simulink model "star_measurement_model"  (R2025a)
settings: Solver=FixedStepAuto  StartTime=0.0  StopTime=5000  FixedStep=0.5  RelTol=1e-4
model mask{star=star}
model workspace (MAT data in the model file):
  star = 0
values from neighbouring files (symbols this model uses):
  m = size(A, 2)    [wheel_analysis.m]
  s = sign(h_bias)    [min_h.m]
  star_Ts = star.Ts    [orbit_params.m]
  Ts = 0.1    [orbit_params.m]    (also in untitled2.m = 0.005)
undefined symbols (not defined in the file or in its folder): earth, sigma_u, sigma_v
libraries: simulink x9, dspmathops x5, aerolibutil x4, utilities x2, simulink_extras x1
settings Model: ParameterArgumentNames=star  Creator=OlguPilav  LastModifiedBy=OlguPilav
settings DataIOCC: SaveOutput=off  SaveTime=off

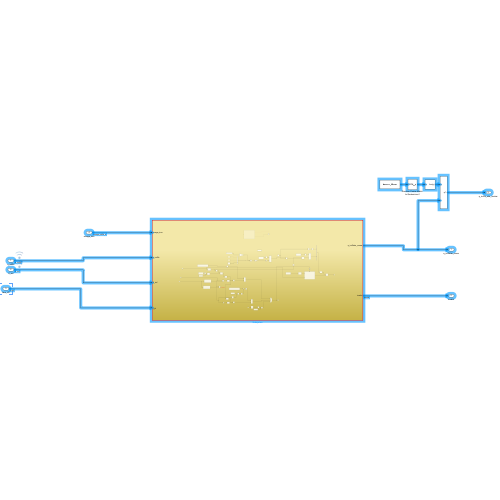
[thumbnail: Simulink's stored preview of the top-level diagram]
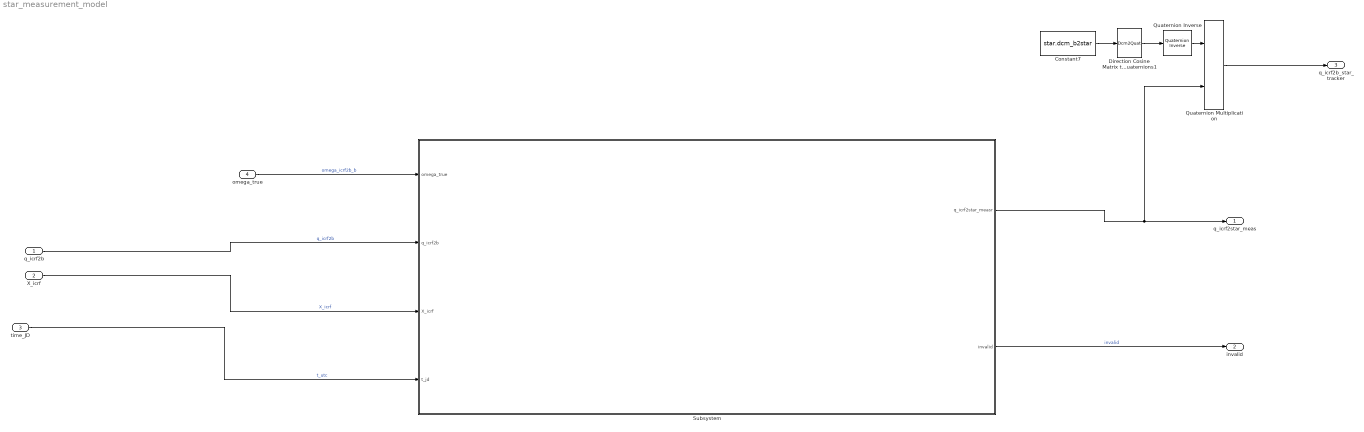
== system star_measurement_model ==
  q_icrf2b : Inport  OutDataTypeStr=double  PortDimensions=[4 1]  SampleTime=0
  X_icrf : Inport  Port=2  OutDataTypeStr=double  PortDimensions=3  SampleTime=0
  time_JD : Inport  Port=3  OutDataTypeStr=double  PortDimensions=1  SampleTime=0
  omega_true : Inport  Port=4  OutDataTypeStr=double  PortDimensions=3  SampleTime=0
  Constant7 : Constant  Value=star.dcm_b2star
  Direction Cosine Matrix to Quaternions1 : Dcm2Quat
  Quaternion Inverse : aerolibutil/Quaternion Inverse
  Quaternion Multiplication : aerolibutil/Quaternion Multiplication
  Subsystem : Subsystem  TreatAsAtomicUnit=on  SystemSampleTime=star_Ts
  q_icrf2star_meas : Outport  OutDataTypeStr=double  PortDimensions=4  SampleTime=[0.5,0]
  invalid : Outport  Port=2  OutDataTypeStr=boolean  PortDimensions=1  SampleTime=[0.5,0]
  q_icrf2b_star_tracker : Outport  Port=3  OutDataTypeStr=double  PortDimensions=4  SampleTime=[0.5,0]
  wires:
  q_icrf2b/1 -> Subsystem/2(q_icrf2b)  "q_icrf2b"
  X_icrf/1 -> Subsystem/3(X_icrf)  "X_icrf"
  time_JD/1 -> Subsystem/4(t_jd)  "t_utc"
  Subsystem/1(q_icrf2star_measr) -> q_icrf2star_meas/1, Quaternion Multiplication/2
  omega_true/1 -> Subsystem/1(omega_true)  "omega_icrf2b_b"
  Subsystem/2(invalid) -> invalid/1  "invalid"
  Quaternion Multiplication/1 -> q_icrf2b_star_tracker/1
  Constant7/1 -> Direction Cosine Matrix to Quaternions1/1
  Quaternion Inverse/1 -> Quaternion Multiplication/1
  Direction Cosine Matrix to Quaternions1/1 -> Quaternion Inverse/1

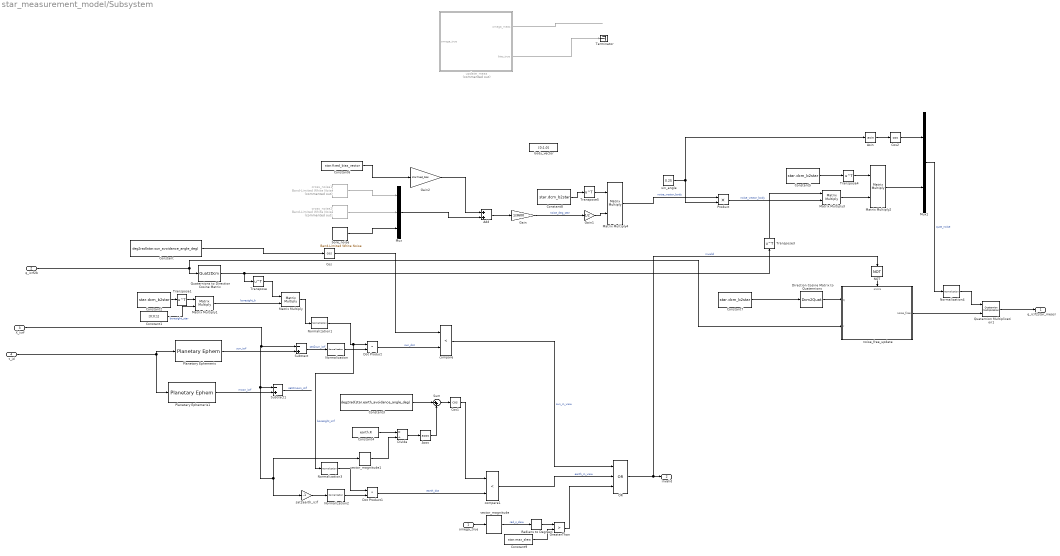
== system star_measurement_model/Subsystem ==
  omega_true : Inport
  q_icrf2b : Inport  Port=2
  X_icrf : Inport  Port=3
  t_jd : Inport  Port=4
  Acos : Trigonometry  Operator=acos
  Add : Sum
  Asin : Trigonometry  Operator=asin
  Constant : Constant  Value=deg2rad(star.sun_avoidance_angle_deg)
  Constant1 : Constant  Value=[0;0;1]
  Constant{2,5,7..8} (4 alike) : Constant  Value=star.dcm_b2star
  Constant3 : Constant  Value=deg2rad(star.earth_avoidance_angle_deg)
  Constant4 : Constant  Value=earth.R
  Constant6 : Constant  Value=star.fixed_bias_vector
  Constant9 : Constant  Value=star.max_slew
  Cos : Trigonometry  Operator=cos
  Cos1 : Trigonometry  Operator=cos
  Cos2 : Trigonometry  Operator=cos
  Direction Cosine Matrix to Quaternions : Dcm2Quat
  Divide : Product  Inputs=*/
  Dot Product : DotProduct  OutDataTypeStr=Inherit: Inherit via internal rule
  Dot Product1 : DotProduct  OutDataTypeStr=Inherit: Inherit via internal rule
  Gain : Gain  Gain=1/3600
  Gain1 : Gain  Gain=1/2
  Gain2 : Gain  Gain=star.fixed_bias
  GreaterThan : RelationalOperator  Operator=>  OutDataTypeStr=boolean  RndMeth=Simplest  InputSameDT=off
  Matrix Multiply{,1..4} (5 alike) : Product  Multiplication=Matrix(*)
  Mux : Mux  Inputs=3
  Mux1 : Mux  Inputs=2
  NOT : Logic  Operator=NOT  IconShape=distinctive  AllPortsSameDT=off  OutDataTypeStr=boolean
  Normalization{,1..4} (5 alike) : dspmathops/Normalization  NormType=2-norm  Bias=1e-10  NormOver=Each column  Dimension=1  roundingMode=Floor  overflowMode=off  accumDataTypeStr=Inherit: Same as product output  accumLastDataTypeStr=Inherit: Same as product output  outputDataTypeStr=Inherit: Same as product output  outputMin=[]  outputMax=[]  outputLastDataTypeStr=Inherit: Same as product output
  OR : Logic  Operator=OR  Inputs=3  IconShape=distinctive  AllPortsSameDT=off  OutDataTypeStr=boolean
  Planetary Ephemeris : PlanetaryEphem  units=m,m/s  target=Sun  outputVelocity=off
  Planetary Ephemeris1 : PlanetaryEphem  units=m,m/s  outputVelocity=off
  Product : Product
  Quaternion Multiplication1 : aerolibutil/Quaternion Multiplication
  Quaternions to Direction Cosine Matrix : Quat2Dcm
  Radians to Degrees : simulink_extras/Transformations/Radians to Degrees
  Subtract : Sum  Inputs=-+
  Subtract1 : Sum  Inputs=-+
  Sum : Sum  Inputs=|++
  Terminator : Terminator
  Transpose{,1,3..5} (5 alike) : Math  Operator=transpose
  body_vector : Constant  Value=[0;1;0]
  bore_noise : simulink/Sources/Band-Limited White Noise  Cov=1  Ts=star_Ts  seed=[678]
  compare : RelationalOperator  Operator=<  OutDataTypeStr=boolean  RndMeth=Simplest  InputSameDT=off
  compare1 : RelationalOperator  Operator=<  OutDataTypeStr=boolean  RndMeth=Simplest  InputSameDT=off
  cross_noise1 : simulink/Sources/Band-Limited White Noise  Commented=on  Cov=[star.sigma_cross^2 * star.Ts]  Ts=star_Ts  seed=[394]
  cross_noise2 : simulink/Sources/Band-Limited White Noise  Commented=on  Cov=[star.sigma_cross^2 * star.Ts]  Ts=star_Ts  seed=[34]
  noise_free_update : Subsystem
  sat2earth_icrf : Gain  Gain=-1
  sin_angle : Constant  Value=0.25
  update_meas : Subsystem  Commented=on  TreatAsAtomicUnit=on  SystemSampleTime=Ts
  vector_magnitude : utilities/vector_magnitude
  vector_magnitude1 : utilities/vector_magnitude
  q_icrf2star_measr : Outport
  invalid : Outport  Port=2
  wires:
  Constant9/1 -> GreaterThan/2
  GreaterThan/1 -> OR/3
  NOT/1 -> noise_free_update/Enable
  noise_free_update/1(noise_free) -> Quaternion Multiplication1/2
  Direction Cosine Matrix to Quaternions/1 -> noise_free_update/1(q)
  Radians to Degrees/1 -> GreaterThan/1
  vector_magnitude/1 -> Radians to Degrees/1  "rad_s_slew"
  Gain2/1 -> Add/1
  Constant6/1 -> Gain2/1
  Add/1 -> Gain/1
  Transpose5/1 -> Matrix Multiply4/1
  Constant8/1 -> Transpose5/1
  Matrix Multiply2/1 -> Mux1/2
  Transpose4/1 -> Matrix Multiply2/1
  Constant5/1 -> Transpose4/1
  Asin/1 -> Cos2/1
  sin_angle/1 -> Asin/1, Product/2
  Matrix Multiply4/1 -> Product/1  "noise_vector_body"
  Quaternion Multiplication1/1 -> q_icrf2star_measr/1
  Transpose3/1 -> Matrix Multiply3/1
  Matrix Multiply3/1 -> Matrix Multiply2/2
  Normalization4/1 -> Quaternion Multiplication1/1
  Product/1 -> Matrix Multiply3/2  "noise_vector_body"
  Subtract1/1 -> ?  "sat2moon_icrf"
  Gain/1 -> Gain1/1  "noise_deg_star"
  cross_noise1/1 -> Mux/1
  Dot Product1/1 -> compare1/2  "earth_dot"
  OR/1 -> invalid/1, NOT/1  "invalid"
  Normalization2/1 -> Dot Product1/2
  Normalization3/1 -> Dot Product1/1
  Transpose1/1 -> Matrix Multiply1/1
  Mux/1 -> Add/2
  Constant4/1 -> Divide/1
  Mux1/1 -> Normalization4/1  "quat_noise"
  Constant3/1 -> Sum/1
  Matrix Multiply1/1 -> Matrix Multiply/2  "boresight_b"
  vector_magnitude1/1 -> Divide/2
  Constant/1 -> Cos/1
  cross_noise2/1 -> Mux/2
  t_jd/1 -> Planetary Ephemeris1/1, Planetary Ephemeris/1
  Divide/1 -> Acos/1
  Constant7/1 -> Direction Cosine Matrix to Quaternions/1
  Matrix Multiply/1 -> Normalization1/1
  q_icrf2b/1 -> Quaternions to Direction Cosine Matrix/1, noise_free_update/2(r)
  compare1/1 -> OR/2  "earth_in_view"
  Cos/1 -> compare/1
  compare/1 -> OR/1  "sun_in_view"
  Transpose/1 -> Matrix Multiply/1
  Subtract/1 -> Normalization/1  "sat2sun_icrf"
  Acos/1 -> Sum/2
  omega_true/1 -> vector_magnitude/1
  Normalization/1 -> Dot Product/2
  Cos1/1 -> compare1/1
  Quaternions to Direction Cosine Matrix/1 -> Transpose/1, Transpose3/1
  Constant2/1 -> Transpose1/1
  update_meas/2(bias_true) -> Terminator/1
  Planetary Ephemeris1/1 -> Subtract1/2  "moon_icrf"
  Normalization1/1 -> Dot Product/1, Normalization3/1  "boresight_icrf"
  update_meas/1(omega_meas) -> ?
  sat2earth_icrf/1 -> Normalization2/1
  Dot Product/1 -> compare/2  "sun_dot"
  Cos2/1 -> Mux1/1
  X_icrf/1 -> Subtract/1, Subtract1/1, sat2earth_icrf/1, vector_magnitude1/1
  Sum/1 -> Cos1/1
  Planetary Ephemeris/1 -> Subtract/2  "sun_icrf"
  Constant1/1 -> Matrix Multiply1/2  "boresight_star"
  bore_noise/1 -> Mux/3
  Gain1/1 -> Matrix Multiply4/2

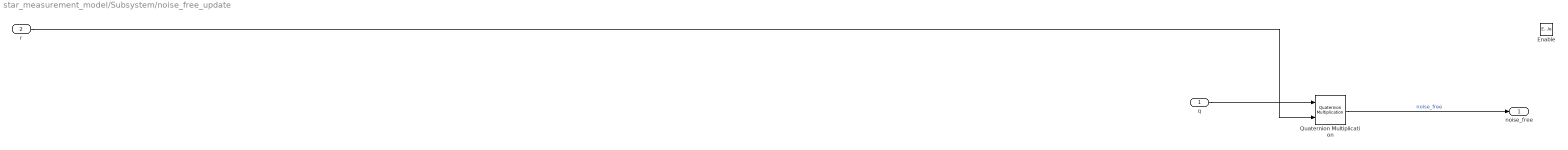
== system star_measurement_model/Subsystem/noise_free_update ==
  q : Inport
  r : Inport  Port=2
  Enable : EnablePort
  Quaternion Multiplication : aerolibutil/Quaternion Multiplication
  noise_free : Outport
  wires:
  r/1 -> Quaternion Multiplication/2
  q/1 -> Quaternion Multiplication/1
  Quaternion Multiplication/1 -> noise_free/1  "noise_free"

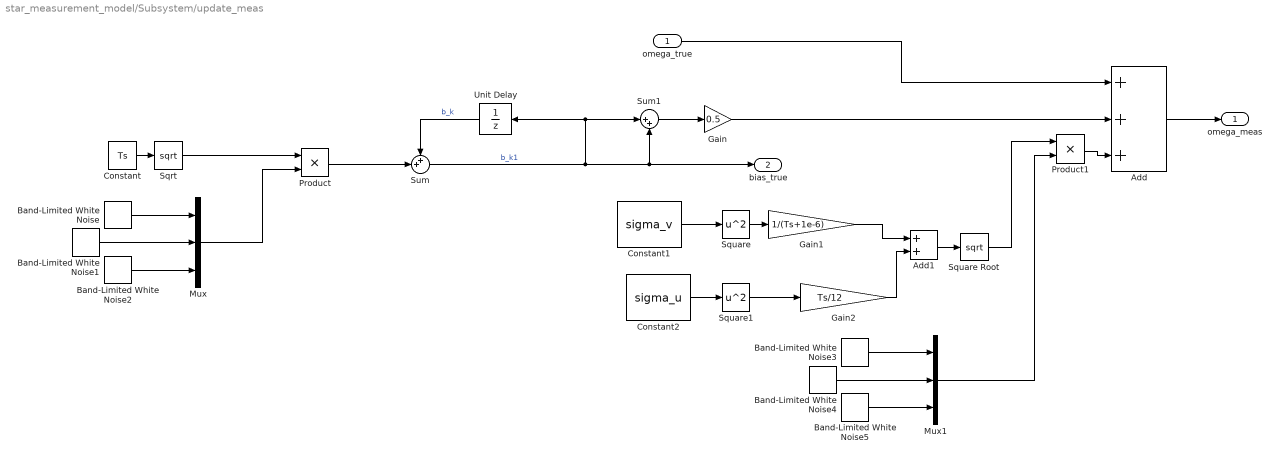
== system star_measurement_model/Subsystem/update_meas ==
  omega_true : Inport
  Add : Sum  Inputs=+++
  Add1 : Sum
  Band-Limited White Noise : simulink/Sources/Band-Limited White Noise  Cov=[Ts * sigma_u]  Ts=Ts  seed=[23341]
  Band-Limited White Noise1 : simulink/Sources/Band-Limited White Noise  Cov=[Ts * sigma_u]  Ts=Ts  seed=[2335341]
  Band-Limited White Noise2 : simulink/Sources/Band-Limited White Noise  Cov=[Ts * sigma_u]  Ts=Ts  seed=[231]
  Band-Limited White Noise3 : simulink/Sources/Band-Limited White Noise  Cov=[Ts * sigma_u]  Ts=Ts  seed=[23341]
  Band-Limited White Noise4 : simulink/Sources/Band-Limited White Noise  Cov=[Ts]  Ts=Ts  seed=[2335341]
  Band-Limited White Noise5 : simulink/Sources/Band-Limited White Noise  Cov=[Ts * sigma_u]  Ts=Ts  seed=[231]
  Constant : Constant  Value=Ts
  Constant1 : Constant  Value=sigma_v
  Constant2 : Constant  Value=sigma_u
  Gain : Gain  Gain=0.5
  Gain1 : Gain  Gain=1/(Ts+1e-6)
  Gain2 : Gain  Gain=Ts/12
  Mux : Mux  Inputs=3
  Mux1 : Mux  Inputs=3
  Product : Product
  Product1 : Product
  Sqrt : Sqrt
  Square : Math  Operator=square
  Square Root : Sqrt
  Square1 : Math  Operator=square
  Sum : Sum  Inputs=++|
  Sum1 : Sum  Inputs=|++
  Unit Delay : UnitDelay  SampleTime=-1  HasFrameUpgradeWarning=on
  omega_meas : Outport
  bias_true : Outport  Port=2
  wires:
  omega_true/1 -> Add/1
  Square Root/1 -> Product1/1
  Add1/1 -> Square Root/1
  Gain2/1 -> Add1/2
  Gain1/1 -> Add1/1
  Square1/1 -> Gain2/1
  Constant2/1 -> Square1/1
  Square/1 -> Gain1/1
  Constant1/1 -> Square/1
  Product1/1 -> Add/3
  Band-Limited White Noise3/1 -> Mux1/1
  Band-Limited White Noise5/1 -> Mux1/3
  Mux1/1 -> Product1/2
  Band-Limited White Noise4/1 -> Mux1/2
  Gain/1 -> Add/2
  Add/1 -> omega_meas/1
  Sum1/1 -> Gain/1
  Mux/1 -> Product/2
  Sqrt/1 -> Product/1
  Product/1 -> Sum/2
  Band-Limited White Noise/1 -> Mux/1
  Band-Limited White Noise1/1 -> Mux/2
  Band-Limited White Noise2/1 -> Mux/3
  Constant/1 -> Sqrt/1
  Unit Delay/1 -> Sum/1  "b_k"
  Sum/1 -> Sum1/2, bias_true/1, Unit Delay/1, Sum1/1  "b_k1"
